simulink model "Speed_Control"  (R2016a)
settings: Solver=VariableStepAuto  StartTime=0.0  StopTime=10.0  RelTol=1e-3
libraries: simulink x2
settings Model: Creator=Pection  LastModifiedBy=Pection

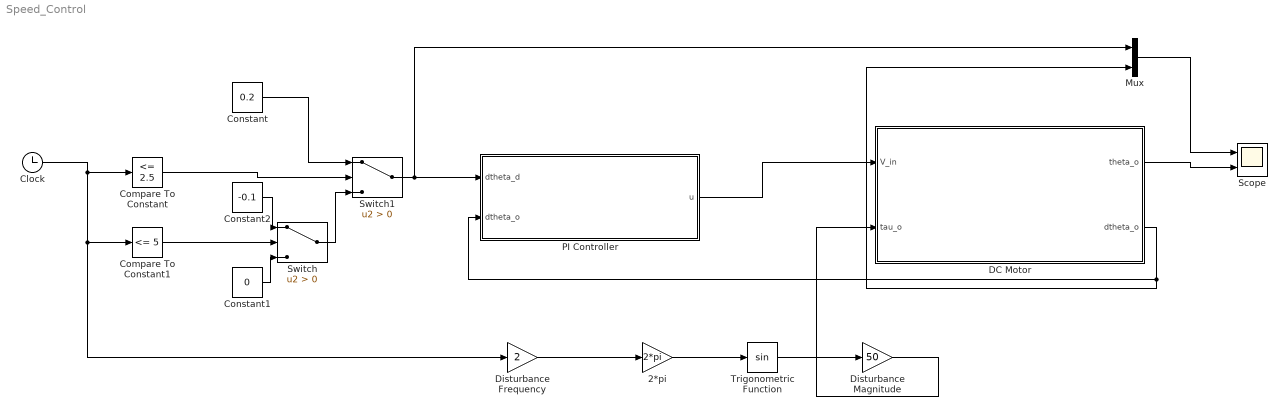
== system Speed_Control ==
  2*pi : Gain  Gain=2*pi
  Clock : Clock
  Compare To Constant : simulink/Logic and Bit Operations/Compare To Constant  relop=<=  const=2.5  OutDataTypeStr=boolean
  Compare To Constant1 : simulink/Logic and Bit Operations/Compare To Constant  relop=<=  const=5  OutDataTypeStr=boolean
  Constant : Constant  Value=0.2
  Constant1 : Constant  Value=0
  Constant2 : Constant  Value=-0.1
  DC Motor : Subsystem  mask(Dc_motor){j_m=2, B_m=0.1, rg=20, L=0.1, K_b=1, K_m=10, R=10}
      mask prompts: j_m "Motor Inertial"; B_m "Damp"; rg "Gear Ratio"; L "Inductor"; K_b "Kb"; K_m "Km"; R "Resistance"
      mask help: Homework
  Disturbance Frequency : Gain  Gain=2
  Disturbance Magnitude : Gain  Gain=50
  Mux : Mux  Inputs=2
  PI Controller : Subsystem  mask{K_i=70, K_p=150}
      mask prompts: K_i "Ki"; K_p "Kp"
  Scope : Scope  NumInputPorts=2
  Switch : Switch  Criteria=u2 > Threshold
  Switch1 : Switch  Criteria=u2 > Threshold
  Trigonometric Function : Trigonometry
  wires:
  Constant2/1 -> Switch/1
  Constant1/1 -> Switch/3
  Compare To Constant1/1 -> Switch/2
  Switch/1 -> Switch1/3
  Switch1/1 -> Mux/1, PI Controller/1(dtheta_d)
  Compare To Constant/1 -> Switch1/2
  Constant/1 -> Switch1/1
  Clock/1 -> Disturbance Frequency/1, Compare To Constant1/1, Compare To Constant/1
  Disturbance Frequency/1 -> 2*pi/1
  2*pi/1 -> Trigonometric Function/1
  Trigonometric Function/1 -> Disturbance Magnitude/1
  Disturbance Magnitude/1 -> DC Motor/2(tau_o)
  PI Controller/1(u) -> DC Motor/1(V_in)
  DC Motor/2(dtheta_o) -> Mux/2, PI Controller/2("dtheta_o ")
  DC Motor/1("theta_o ") -> Scope/2
  Mux/1 -> Scope/1

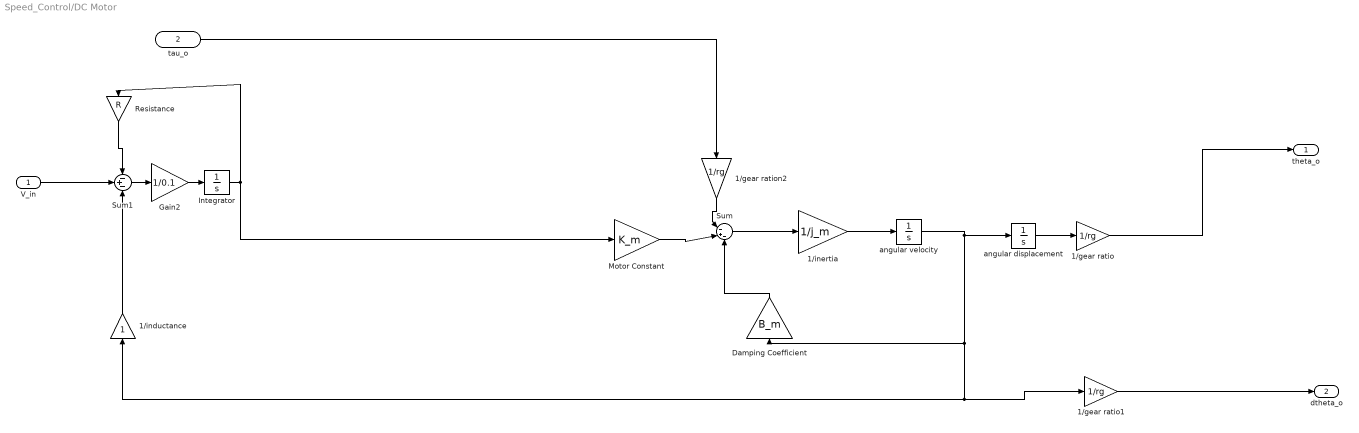
== system Speed_Control/DC Motor ==
  V_in : Inport
  tau_o : Inport  Port=2
  1/gear ratio : Gain  Gain=1/rg
  1/gear ratio1 : Gain  Gain=1/rg
  1/gear ration2 : Gain  Gain=1/rg
  1/inductance : Gain
  "1/inertia " : Gain  Gain=1/j_m
  Damping Coefficient : Gain  Gain=B_m
  Gain2 : Gain  Gain=1/0.1
  Integrator : Integrator
  Motor Constant : Gain  Gain=K_m
  "Resistance " : Gain  Gain=R
  Sum : Sum  Inputs=|-+-
  Sum1 : Sum  Inputs=-+-
  angular displacement : Integrator
  "angular velocity " : Integrator
  "theta_o " : Outport
  dtheta_o : Outport  Port=2
  wires:
  angular displacement/1 -> 1/gear ratio/1
  Sum/1 -> "1/inertia "/1
  "Resistance "/1 -> Sum1/1
  V_in/1 -> Sum1/2
  1/inductance/1 -> Sum1/3
  1/gear ratio/1 -> "theta_o "/1
  Gain2/1 -> Integrator/1
  Sum1/1 -> Gain2/1
  1/gear ratio1/1 -> dtheta_o/1
  "angular velocity "/1 -> 1/inductance/1, 1/gear ratio1/1, Damping Coefficient/1, angular displacement/1
  1/gear ration2/1 -> Sum/1
  tau_o/1 -> 1/gear ration2/1
  "1/inertia "/1 -> "angular velocity "/1
  Damping Coefficient/1 -> Sum/3
  Motor Constant/1 -> Sum/2
  Integrator/1 -> Motor Constant/1, "Resistance "/1

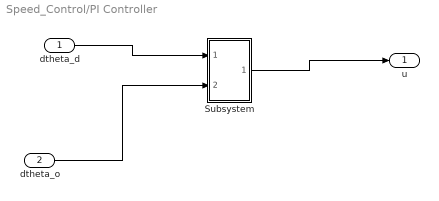
== system Speed_Control/PI Controller ==
  dtheta_d : Inport
  "dtheta_o " : Inport  Port=2
  Subsystem : Subsystem
  u : Outport
  wires:
  dtheta_d/1 -> Subsystem/1(v_d)
  "dtheta_o "/1 -> Subsystem/2("dtheta_o ")
  Subsystem/1(Out1) -> u/1

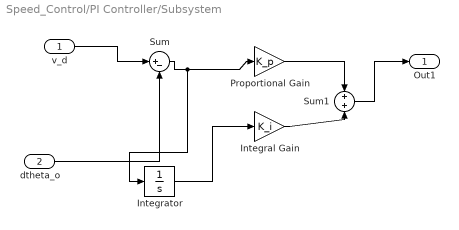
== system Speed_Control/PI Controller/Subsystem ==
  v_d : Inport
  "dtheta_o " : Inport  Port=2
  Integral Gain : Gain  Gain=K_i
  Integrator : Integrator
  "Proportional Gain " : Gain  Gain=K_p
  Sum : Sum  Inputs=|+-
  Sum1 : Sum
  Out1 : Outport
  wires:
  Integrator/1 -> Integral Gain/1
  v_d/1 -> Sum/1
  Sum/1 -> Integrator/1, "Proportional Gain "/1
  "Proportional Gain "/1 -> Sum1/1
  Sum1/1 -> Out1/1
  Integral Gain/1 -> Sum1/2
  "dtheta_o "/1 -> Sum/2
